simulink model "pb_truncation"  (R2014a)
settings: Solver=ode45  StartTime=0.0  StopTime=10  RelTol=1e-3
libraries: truetime x5
settings Model: Creator=Jiangtao He  LastModifiedBy=Jiangtao He

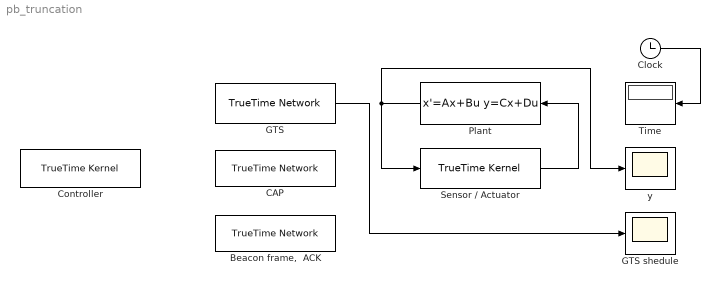
== system pb_truncation ==
  "Beacon frame,  ACK" : truetime/TrueTime Network  nwtype=CSMA/AMP (CAN)  nwnbr=3  nnodes=2  rate=250000  minsize=960  lossprob=0  seed=0  bandwidths=[0.5 0.5]  slotsize=512  schedule=[1 1 2]  memsize=80000  buftype=Common buffer  overflow=Retransmit  dynSchedule=0  miniSlotSize=0  NIT=0  QSortMode=FIFO  sync=0  irtSchedule=0  nrtLength=0  nodeGraph=0  scheduleoutput=off
  CAP : truetime/TrueTime Network  nwtype=CSMA/AMP (CAN)  nwnbr=2  nnodes=2  rate=10000000  minsize=512  lossprob=0.5  seed=0  bandwidths=[0.5 0.5]  slotsize=512  schedule=[1 1 2]  memsize=80000  buftype=Common buffer  overflow=Retransmit  dynSchedule=0  miniSlotSize=0  NIT=0  QSortMode=FIFO  sync=0  irtSchedule=0  nrtLength=0  nodeGraph=0  scheduleoutput=off
  Clock : Clock
  Controller : truetime/TrueTime Kernel  sfun=con_init  args=12.5  ninputsoutputs=[0 0]  ntriggers=0  trigtype=falling  nwnodenbr=[1 2;2 2;3 2]  clockoffsetdrift=[0 0]  schedoutput=off  battery=off  poweroutput=off  label=1: 2\n2: 2\n3: 2
  GTS : truetime/TrueTime Network  nwtype=CSMA/AMP (CAN)  nwnbr=1  nnodes=2  rate=10000000  minsize=512  lossprob=0.02  seed=0  bandwidths=[0.5 0.5]  slotsize=512  schedule=[1 1 2]  memsize=80000  buftype=Common buffer  overflow=Retransmit  dynSchedule=0  miniSlotSize=0  NIT=0  QSortMode=FIFO  sync=0  irtSchedule=0  nrtLength=0  nodeGraph=0  scheduleoutput=on
  GTS shedule : Scope
      settings: ShowLegends=on  TimeRange=10  YMin=1  YMax=3
  Plant : StateSpace  A=[0 1;9.8 0]  B=[0;-0.3333]  C=[1 0;0 1]  D=[0;0]  X0=[0;-90]
  "Sensor / Actuator " : truetime/TrueTime Kernel  sfun=S_A_init  args=0.04  ninputsoutputs=[2 1]  ntriggers=0  trigtype=falling  nwnodenbr=[1 1;2 1;3 1]  clockoffsetdrift=[0 0]  schedoutput=off  battery=off  poweroutput=off  label=1: 1\n2: 1\n3: 1
  Time : Display
  y : Scope
      settings: ShowLegends=on  TimeRange=10  YMin=1  YMax=2.5
  wires:
  Plant/1 -> "Sensor / Actuator "/1, y/1
  "Sensor / Actuator "/1 -> Plant/1
  GTS/1 -> GTS shedule/1
  Clock/1 -> Time/1
